simulink subsystem "OpenDifferential"  (R2025a)
settings: Solver=VariableStepAuto  StartTime=0.0  StopTime=10.0  RelTol=1e-3
libraries: autolibshareddiff x1
settings Model: Creator=The MathWorks, Inc.  LastModifiedBy=The MathWorks, Inc.
settings RTWCC: GPUComputeCapability=3.5

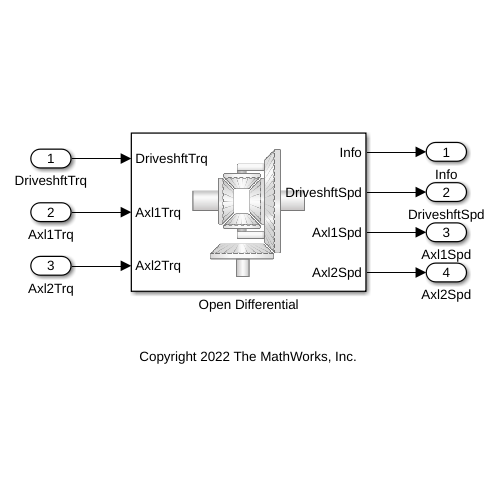
[thumbnail: Simulink's stored preview of the top-level diagram]
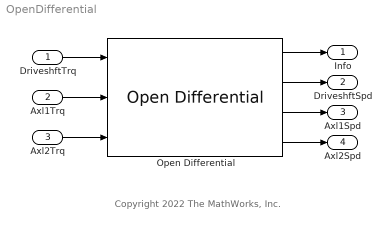
== system OpenDifferential ==
  note: Copyright 2022 The MathWorks, Inc.
  DriveshftTrq : Inport
  Axl1Trq : Inport  Port=2
  Axl2Trq : Inport  Port=3
  Open Differential : autolibshareddiff/Open Differential  VariantControl=Open Differential  DiffEffModelPopup=Constant  InterpMethod=Linear point-slope  extTamb=off  shaftSwitchMask=To the left of center-line  Ndiff=PlntDiffrntlRatio  Jd=PlntDiffrntlCarrInertia  bd=PlntDiffrntlCarrDamp  Jw1=PlntDiffrntlAxl1Inertia  bw1=PlntDiffrntlAxl1Damp  Jw2=PlntDiffrntlAxl2Inertia  bw2=PlntDiffrntlAxl2Damp  omegaw1o=PlntDiffrntlAxl1InitVel  omegaw2o=PlntDiffrntlAxl2InitVel  eta=PlntDiffrntlEff  eta_tbl=PlntDiffrntlEffTbl  Trq_bpts=PlntDiffrntlEffTrqBpt  omega_bpts=PlntDiffrntlEffSpdBpt  Temp_bpts=PlntDiffrntlEffTempBpt  Tamb=EnvAirTemp  maxAbsSpd=5e3  aMode=6
  Info : Outport
  DriveshftSpd : Outport  Port=2
  Axl1Spd : Outport  Port=3
  Axl2Spd : Outport  Port=4
  wires:
  Open Differential/1 -> Info/1
  Open Differential/2 -> DriveshftSpd/1
  Open Differential/3 -> Axl1Spd/1
  Open Differential/4 -> Axl2Spd/1
  DriveshftTrq/1 -> Open Differential/1
  Axl1Trq/1 -> Open Differential/2
  Axl2Trq/1 -> Open Differential/3
